simulink library "FirGeneric"  (R2022b)
settings: Solver=VariableStepAuto  StartTime=0.0  StopTime=10.0  RelTol=1e-3
undefined symbols (not defined in the file or in its folder): Row
libraries: HandyTextFile x9, TuneVar x9, FeaturePath x3, $bdroot x2, TOP x2, RTC x1
settings Model: Creator=fz1054048  LastModifiedBy=jk1043656

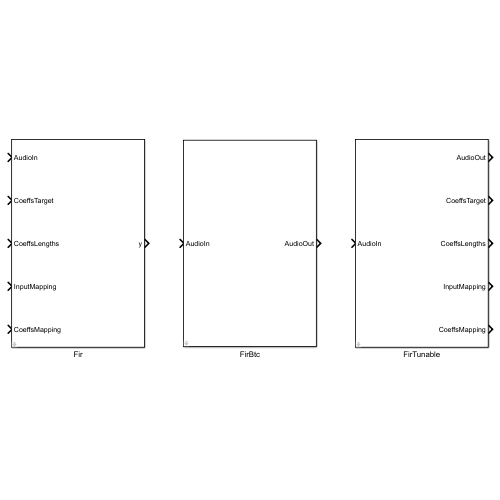
[thumbnail: Simulink's stored preview of the top-level diagram]
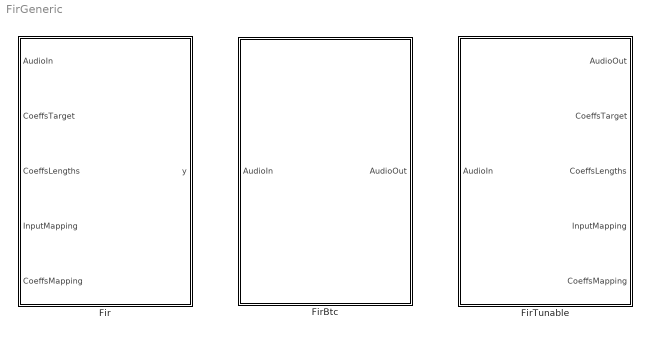
== system FirGeneric ==
  Fir : Subsystem  mask(Blocklib Fir){Config=[], FeatureName=Fir}
      mask prompts: Config "FirConfig"; FeatureName "Feature path name:"
      mask help:
      | For more information, see 'Help'. or run
      | >> help FirConfig
      mask init:
      | blkh=gcbh;
      | Config=BTConfig.Assert(blkh,Config);
      | 
      | Config.Validate();
      | Config.DoMaskInit(blkh);
      mask Help: eval("help FirConfig")
      mask TypeOptions FeatureName: FeaturePath/FeatureName
  FirBtc : Subsystem  mask(Blocklib FirBtc){Config=[], FeatureName=FirBtc}
      mask prompts: Config "FirBtcConfig"; FeatureName "Feature path name:"
      mask help:
      | For more information, see "Help" or run
      | >> help FirBtcConfig
      mask init:
      | blkh=gcbh;
      | Config=BTConfig.Assert(blkh,Config);
      | 
      | Config.Validate();
      | Config.DoMaskInit(blkh);
      mask Help: eval("help FirBtcConfig")
      mask TypeOptions FeatureName: FeaturePath/FeatureName
  FirTunable : Subsystem  mask(Blocklib FirTunable){Config=[], FeatureName=FirTunable}
      mask prompts: Config "FirTunableConfig"; FeatureName "Feature path name:"
      mask help:
      | For more information, see "Help" or run
      | >> help FirConfig
      mask init:
      | blkh=gcbh;
      | Config=BTConfig.Assert(blkh,Config);
      | 
      | Config.Validate();
      | Config.DoMaskInit(blkh);
      mask Help: eval("help FirConfig")
      mask TypeOptions FeatureName: FeaturePath/FeatureName

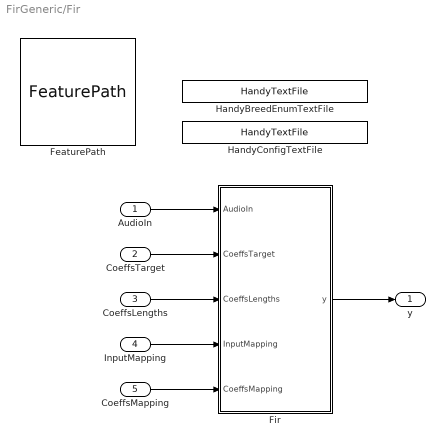
== system FirGeneric/Fir ==
  AudioIn : Inport
  CoeffsTarget : Inport  Port=2
  CoeffsLengths : Inport  Port=3
  InputMapping : Inport  Port=4
  CoeffsMapping : Inport  Port=5
  FeaturePath : FeaturePath/FeaturePath  FeatureName=Fir  IsGroup=off  GroupNumber=-1  IsModule=off  TriggerInit=[-5 -21 110 86]
      settings: SourceProductName=Bose Talaria
  Fir : Subsystem  Variant=on
  HandyBreedEnumTextFile : HandyTextFile/HandyTextFile  TemplateSource=<dialog fields>  FileSuffix=BreedEnum  OpenDialogOnLoad=off  UseThisBlockName=off  AddGrandParentNamePrefix=off  TheDefaultText=% $(FILENAME) $(PREFIX) $(SUFFIX)  ShowInLibBrowser=on
      settings: SourceProductName=Bose Talaria
  HandyConfigTextFile : HandyTextFile/HandyTextFile  TemplateSource=Config  FileSuffix=File  OpenDialogOnLoad=off  UseThisBlockName=off  AddGrandParentNamePrefix=off  TheDefaultText=% $(FILENAME) $(PREFIX) $(SUFFIX)  ShowInLibBrowser=on
      settings: SourceProductName=Bose Talaria
  y : Outport
  wires:
  AudioIn/1 -> Fir/1(AudioIn)
  CoeffsLengths/1 -> Fir/3(CoeffsLengths)
  InputMapping/1 -> Fir/4(InputMapping)
  CoeffsMapping/1 -> Fir/5(CoeffsMapping)
  Fir/1(y) -> y/1
  CoeffsTarget/1 -> Fir/2(CoeffsTarget)

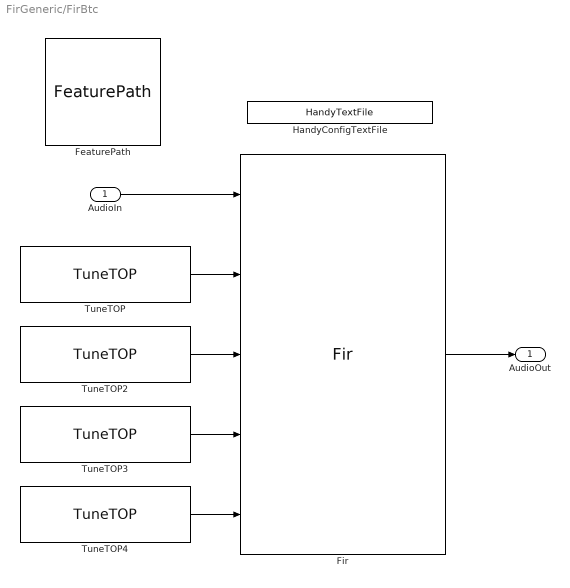
== system FirGeneric/FirBtc ==
  AudioIn : Inport
  FeaturePath : FeaturePath/FeaturePath  FeatureName=FirBtc  IsGroup=off  GroupNumber=-1  IsModule=off  TriggerInit=[-35 -26 80 81]
      settings: SourceProductName=Bose Talaria
  Fir : $bdroot/Fir  Config=Config  FeatureName=Fir
  HandyConfigTextFile : HandyTextFile/HandyTextFile  TemplateSource=Config  FileSuffix=File  OpenDialogOnLoad=off  UseThisBlockName=off  AddGrandParentNamePrefix=off  TheDefaultText=% $(FILENAME) $(PREFIX) $(SUFFIX)  ShowInLibBrowser=on
      settings: SourceProductName=Bose Talaria
  TuneTOP : TuneVar/TuneTOP  TriggerInit=[-60 182 110 238]  TopName=CoeffsTarget  TuneName=CoeffsTarget  DataTypeOut=single  TunabilityNumber=1  MinValue=[]  MaxValue=[]  BankNumber=Config.BankNumber  PreOverlay=false  PostOverlay=Config.PostOverlayRequired  UseSameName=on  MaskValue=Config.TuneVarCoeffsTarget
      settings: SourceProductName=Bose Talaria
  TuneTOP2 : TuneVar/TuneTOP  TriggerInit=[-60 262 110 318]  TopName=CoeffsLengths  TuneName=CoeffsLengths  DataTypeOut=uint32  TunabilityNumber=1  MinValue=[]  MaxValue=[]  BankNumber=0  PreOverlay=false  PostOverlay=Config.PostOverlayRequired  UseSameName=on  MaskValue=Config.TuneVarCoeffsLengths
      settings: SourceProductName=Bose Talaria
  TuneTOP3 : TuneVar/TuneTOP  TriggerInit=[-60 342 110 398]  TopName=InputMapping  TuneName=InputMapping  DataTypeOut=uint32  TunabilityNumber=1  MinValue=[]  MaxValue=[]  BankNumber=0  PreOverlay=false  PostOverlay=Config.PostOverlayRequired  UseSameName=on  MaskValue=Config.TuneVarInputMapping
      settings: SourceProductName=Bose Talaria
  TuneTOP4 : TuneVar/TuneTOP  TriggerInit=[-60 422 110 478]  TopName=CoeffsMapping  TuneName=CoeffsMapping  DataTypeOut=uint32  TunabilityNumber=1  MinValue=[]  MaxValue=[]  BankNumber=0  PreOverlay=false  PostOverlay=Config.PostOverlayRequired  UseSameName=on  MaskValue=Config.TuneVarCoeffsMapping
      settings: SourceProductName=Bose Talaria
  AudioOut : Outport
  wires:
  Fir/1 -> AudioOut/1
  TuneTOP4/1 -> Fir/5
  AudioIn/1 -> Fir/1
  TuneTOP/1 -> Fir/2
  TuneTOP2/1 -> Fir/3
  TuneTOP3/1 -> Fir/4

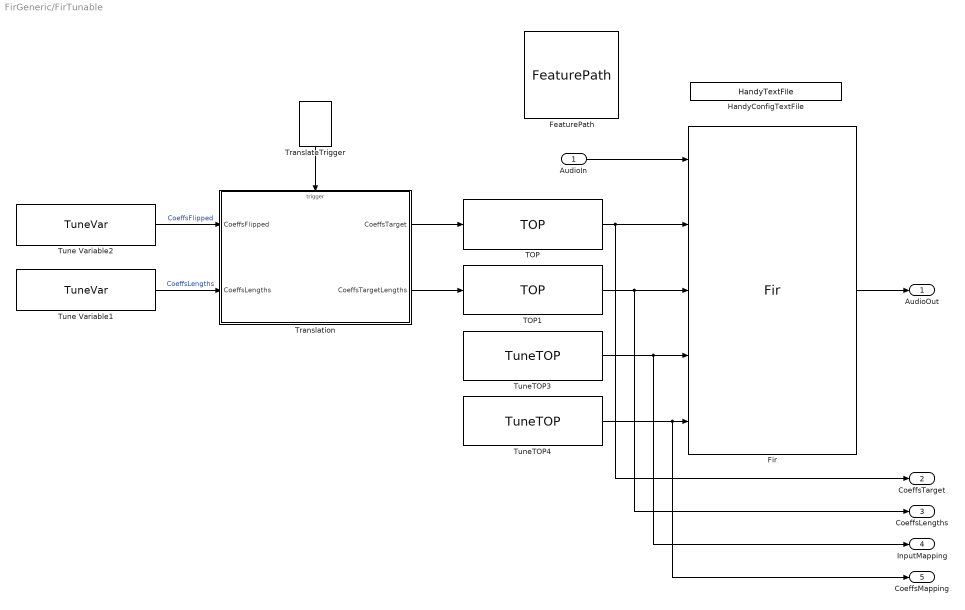
== system FirGeneric/FirTunable ==
  AudioIn : Inport
  FeaturePath : FeaturePath/FeaturePath  FeatureName=FirTunable  IsGroup=off  GroupNumber=-1  IsModule=off  TriggerInit=[-35 -26 80 81]
      settings: SourceProductName=Bose Talaria
  Fir : $bdroot/Fir  Config=Config  FeatureName=Fir
  HandyConfigTextFile : HandyTextFile/HandyTextFile  TemplateSource=Config  FileSuffix=File  OpenDialogOnLoad=off  UseThisBlockName=off  AddGrandParentNamePrefix=off  TheDefaultText=% $(FILENAME) $(PREFIX) $(SUFFIX)  ShowInLibBrowser=on
      settings: SourceProductName=Bose Talaria
  TOP : TOP/TOP  TriggerInit=[-110 180 60 240]  TopName=CoeffsTarget  DataTypeOut=single  BankNumber=Config.BankNumber  PreOverlay=false  PostOverlay=Config.PostOverlayRequired  CompatibilityString=Config.Breed  Role=Automatic
      settings: SourceProductName=Bose Talaria
  TOP1 : TOP/TOP  TriggerInit=[-110 260 60 320]  TopName=CoeffsLengths  DataTypeOut=uint32  BankNumber=0  PreOverlay=false  PostOverlay=Config.PostOverlayRequired  CompatibilityString=Config.Breed  Role=Automatic
      settings: SourceProductName=Bose Talaria
  TranslateTrigger : TuneVar/TranslateTrigger  TriggerInit=[-309 60 -271 115]
      settings: SourceProductName=Bose Talaria
  Translation : MATLAB Function  TreatAsAtomicUnit=on  mask{Breed=Config.Breed, FrameSize=Config.FrameSize, MaxAvgCoeffLength=Config.MaxAvgCoeffLength, NumFilters=Config.NumFilters}
  Tune Variable1 : TuneVar/TuneVar  TuneName=CoeffsLengths  SpecifyMaxSize=off  VariableDim=1 (Row)  MaxSize=[1 1]  TunabilityNumber=1  MinValue=[]  MaxValue=[]  TriggerInit=[-655 265 -485 315]  MaskValue=Config.TuneVarCoeffsLengths
      settings: SourceProductName=Bose Talaria
  Tune Variable2 : TuneVar/TuneVar  TuneName=CoeffsFlipped  SpecifyMaxSize=on  VariableDim=1 (Row)  MaxSize=[Config.MaxAvgCoeffLength*Config.NumFilters,1]  TunabilityNumber=1  MinValue=[]  MaxValue=[]  TriggerInit=[-655 185 -485 235]  MaskValue=Config.TuneVarCoeffsFlipped
      settings: SourceProductName=Bose Talaria
  TuneTOP3 : TuneVar/TuneTOP  TriggerInit=[-110 340 60 400]  TopName=InputMapping  TuneName=InputMapping  DataTypeOut=uint32  TunabilityNumber=1  MinValue=[]  MaxValue=[]  BankNumber=0  PreOverlay=false  PostOverlay=Config.PostOverlayRequired  UseSameName=on  MaskValue=Config.TuneVarInputMapping
      settings: SourceProductName=Bose Talaria
  TuneTOP4 : TuneVar/TuneTOP  TriggerInit=[-110 420 60 480]  TopName=CoeffsMapping  TuneName=CoeffsMapping  DataTypeOut=uint32  TunabilityNumber=1  MinValue=[]  MaxValue=[]  BankNumber=0  PreOverlay=false  PostOverlay=Config.PostOverlayRequired  UseSameName=on  MaskValue=Config.TuneVarCoeffsMapping
      settings: SourceProductName=Bose Talaria
  AudioOut : Outport
  CoeffsTarget : Outport  Port=2
  CoeffsLengths : Outport  Port=3
  InputMapping : Outport  Port=4
  CoeffsMapping : Outport  Port=5
  wires:
  TuneTOP3/1 -> Fir/4, InputMapping/1
  AudioIn/1 -> Fir/1
  TuneTOP4/1 -> Fir/5, CoeffsMapping/1
  Fir/1 -> AudioOut/1
  Translation/2(CoeffsTargetLengths) -> TOP1/1
  TranslateTrigger/1 -> Translation/Trigger
  Tune Variable1/1 -> Translation/2(CoeffsLengths)  "CoeffsLengths"
  Translation/1(CoeffsTarget) -> TOP/1
  Tune Variable2/1 -> Translation/1(CoeffsFlipped)  "CoeffsFlipped"
  TOP1/1 -> Fir/3, CoeffsLengths/1
  TOP/1 -> Fir/2, CoeffsTarget/1

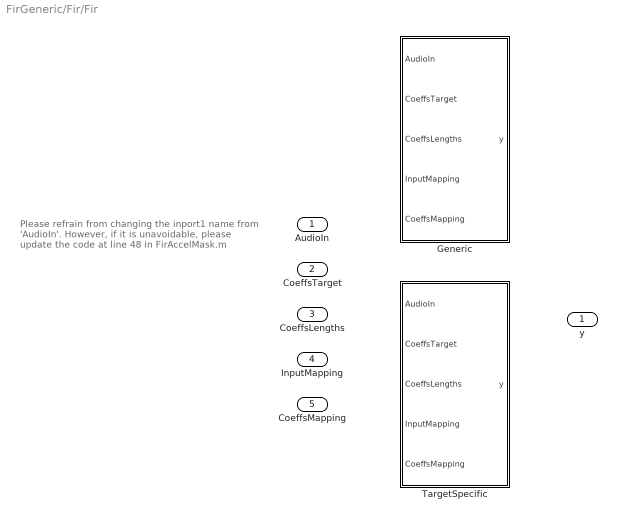
== system FirGeneric/Fir/Fir ==
  note: Please refrain from changing the inport1
      | name from 'AudioIn'. However, if it is
      | unavoidable, please update the code at
      | line 48 in FirAccelMask.m
  AudioIn : Inport
  CoeffsTarget : Inport  Port=2
  CoeffsLengths : Inport  Port=3
  InputMapping : Inport  Port=4
  CoeffsMapping : Inport  Port=5
  Generic : Subsystem  VariantControl=(Config.Breed == AsdHwEnum.Generic)
  TargetSpecific : Subsystem  VariantControl=(default)
  y : Outport

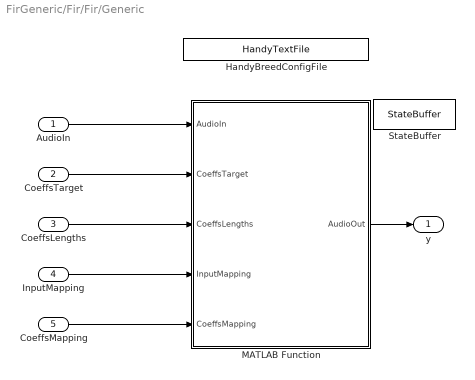
== system FirGeneric/Fir/Fir/Generic ==
  AudioIn : Inport
  CoeffsTarget : Inport  Port=2
  CoeffsLengths : Inport  Port=3
  InputMapping : Inport  Port=4
  CoeffsMapping : Inport  Port=5
  HandyBreedConfigFile : HandyTextFile/HandyTextFile  TemplateSource=<dialog fields>  FileSuffix=BreedConfig  OpenDialogOnLoad=off  UseThisBlockName=off  AddGrandParentNamePrefix=on  TheDefaultText=|  ShowInLibBrowser=on
      | % $(FILENAME) Setup model parameters for each "Init" callback (e.g. update diagram)
      | sample_rate_in_hertz = 44100;
      | frame_size = 32;
      | sysin_channel_count = 2;
      settings: SourceProductName=Bose Talaria
  MATLAB Function : MATLAB Function  TreatAsAtomicUnit=on  mask{FrameSize=Config.FrameSize, NumOutputs=Config.NumOutputs}
  StateBuffer : DataStoreMemory  DataStoreName=StateBuffer  WriteAfterWriteMsg=warning  InitialValue=single(zeros(Config.BreedObj.StateBufferSize,1))  ShowAdditionalParam=off  OutDataTypeStr=single
  y : Outport
  wires:
  AudioIn/1 -> MATLAB Function/1(AudioIn)
  CoeffsTarget/1 -> MATLAB Function/2(CoeffsTarget)
  CoeffsLengths/1 -> MATLAB Function/3(CoeffsLengths)
  InputMapping/1 -> MATLAB Function/4(InputMapping)
  CoeffsMapping/1 -> MATLAB Function/5(CoeffsMapping)
  MATLAB Function/1(AudioOut) -> y/1

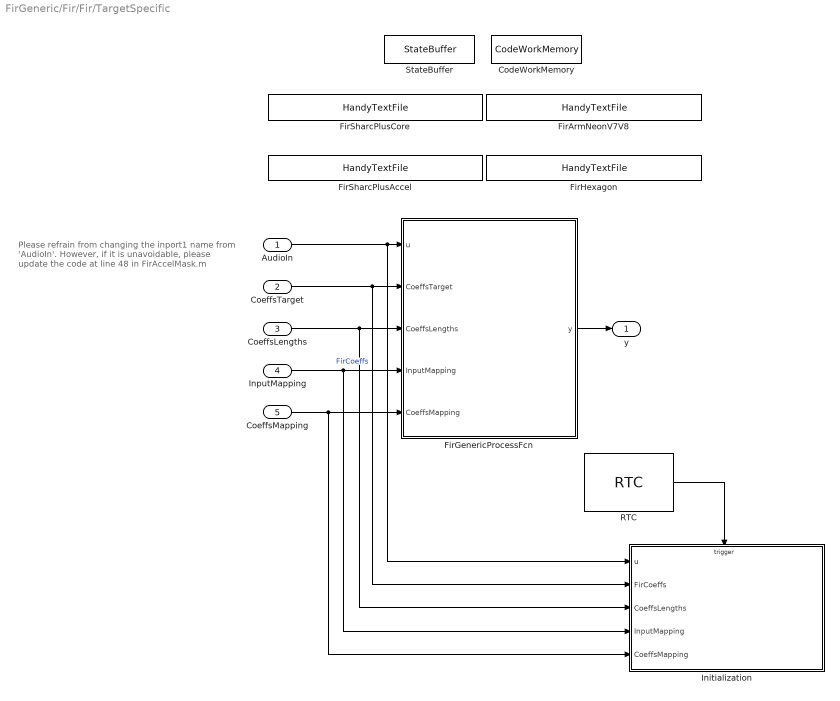
== system FirGeneric/Fir/Fir/TargetSpecific ==
  note: Please refrain from changing the inport1
      | name from 'AudioIn'. However, if it is
      | unavoidable, please update the code at
      | line 48 in FirAccelMask.m
  AudioIn : Inport
  CoeffsTarget : Inport  Port=2
  CoeffsLengths : Inport  Port=3
  InputMapping : Inport  Port=4
  CoeffsMapping : Inport  Port=5
  CodeWorkMemory : DataStoreMemory  DataStoreName=CodeWorkMemory  WriteAfterWriteMsg=warning  InitialValue=uint32(zeros(1,Config.BreedObj.CodeWorkMemorySize))  ShowAdditionalParam=off  OutDataTypeStr=uint32
  FirArmNeonV7V8 : HandyTextFile/HandyTextFile  TemplateSource=<dialog fields>  FileSuffix=BreedConfig  OpenDialogOnLoad=off  UseThisBlockName=on  AddGrandParentNamePrefix=off  TheDefaultText=|  ShowInLibBrowser=on
      | % $(FILENAME) Setup model parameters for each "Init" callback (e.g. update diagram)
      | sample_rate_in_hertz = 44100;
      | frame_size = 32;
      | sysin_channel_count = 2;
      settings: SourceProductName=Bose Talaria
  FirGenericProcessFcn : MATLAB Function  TreatAsAtomicUnit=on  mask{StateBufferSizeSimulation=Config.StateBufferSizeSimulation, Breed=Config.Breed}
  FirHexagon : HandyTextFile/HandyTextFile  TemplateSource=<dialog fields>  FileSuffix=BreedConfig  OpenDialogOnLoad=off  UseThisBlockName=on  AddGrandParentNamePrefix=off  TheDefaultText=|  ShowInLibBrowser=on
      | % $(FILENAME) Setup model parameters for each "Init" callback (e.g. update diagram)
      | sample_rate_in_hertz = 44100;
      | frame_size = 32;
      | sysin_channel_count = 2;
      settings: SourceProductName=Bose Talaria
  FirSharcPlusAccel : HandyTextFile/HandyTextFile  TemplateSource=<dialog fields>  FileSuffix=BreedConfig  OpenDialogOnLoad=off  UseThisBlockName=on  AddGrandParentNamePrefix=off  TheDefaultText=|  ShowInLibBrowser=on
      | % $(FILENAME) Setup model parameters for each "Init" callback (e.g. update diagram)
      | sample_rate_in_hertz = 44100;
      | frame_size = 32;
      | sysin_channel_count = 2;
      settings: SourceProductName=Bose Talaria
  FirSharcPlusCore : HandyTextFile/HandyTextFile  TemplateSource=<dialog fields>  FileSuffix=BreedConfig  OpenDialogOnLoad=off  UseThisBlockName=on  AddGrandParentNamePrefix=off  TheDefaultText=|  ShowInLibBrowser=on
      | % $(FILENAME) Setup model parameters for each "Init" callback (e.g. update diagram)
      | sample_rate_in_hertz = 44100;
      | frame_size = 32;
      | sysin_channel_count = 2;
      settings: SourceProductName=Bose Talaria
  Initialization : Subsystem
  RTC : RTC/RTC  REQ_Priority=RTC_Mask.NormalPriority  RequestAtInit=on  EnableRequest=on  REQElemType1=boolean  REQElemWidth1=1  REQElemInitial1=[]  REQElemType2=uint32  REQElemWidth2=1  REQElemInitial2=[]  REQElemType3=uint32  REQElemWidth3=1  REQElemInitial3=[]  REQElemType4=uint32  REQElemWidth4=1  REQElemInitial4=[]  REQElemType5=uint32  REQElemWidth5=1  REQElemInitial5=[]  REQElemType6=uint32  REQElemWidth6=1  REQElemInitial6=[]  REQElemType7=uint32  REQElemWidth7=1  REQElemInitial7=[]  REQElemType8=uint32  REQElemWidth8=1  REQElemInitial8=[]  REQElemType9=uint32  REQElemWidth9=1  REQElemInitial9=[]  REQElemType10=uint32  REQElemWidth10=1  REQElemInitial10=[]  EnableResponse=off  EnableRSP_StatusIn=off  RSPElemType1=uint32  RSPElemWidth1=1  RSPElemType2=uint32  RSPElemWidth2=1  RSPElemType3=uint32  RSPElemWidth3=1  RSPElemType4=uint32  RSPElemWidth4=1  RSPElemType5=uint32  RSPElemWidth5=1  RSPElemType6=uint32  RSPElemWidth6=1  RSPElemType7=uint32  RSPElemWidth7=1  RSPElemType8=uint32  RSPElemWidth8=1  RSPElemType9=uint32  RSPElemWidth9=1  RSPElemType10=uint32  RSPElemWidth10=1  EnableNotification=off  EnableNTF_PrepTrig=off  NTFElemType1=uint32  NTFElemWidth1=1  NTFElemType2=uint32  NTFElemWidth2=1  NTFElemType3=uint32  NTFElemWidth3=1  NTFElemType4=uint32  NTFElemWidth4=1  NTFElemType5=uint32  NTFElemWidth5=1  NTFElemType6=uint32  NTFElemWidth6=1  NTFElemType7=uint32  NTFElemWidth7=1  NTFElemType8=uint32  NTFElemWidth8=1  NTFElemType9=uint32  NTFElemWidth9=1  NTFElemType10=uint32  NTFElemWidth10=1  MaskMessageName=InitReset
      settings: SourceProductName=Bose Talaria
  StateBuffer : DataStoreMemory  DataStoreName=StateBuffer  WriteAfterWriteMsg=warning  InitialValue=single(zeros(Config.BreedObj.StateBufferSize,1))  ShowAdditionalParam=off  OutDataTypeStr=single
  y : Outport
  wires:
  FirGenericProcessFcn/1(y) -> y/1
  CoeffsTarget/1 -> Initialization/2(FirCoeffs), FirGenericProcessFcn/2(CoeffsTarget)  "FirCoeffs"
  RTC/1 -> Initialization/Trigger
  CoeffsMapping/1 -> Initialization/5(CoeffsMapping), FirGenericProcessFcn/5(CoeffsMapping)
  AudioIn/1 -> Initialization/1(u), FirGenericProcessFcn/1(u)
  InputMapping/1 -> Initialization/4(InputMapping), FirGenericProcessFcn/4(InputMapping)
  CoeffsLengths/1 -> Initialization/3(CoeffsLengths), FirGenericProcessFcn/3(CoeffsLengths)

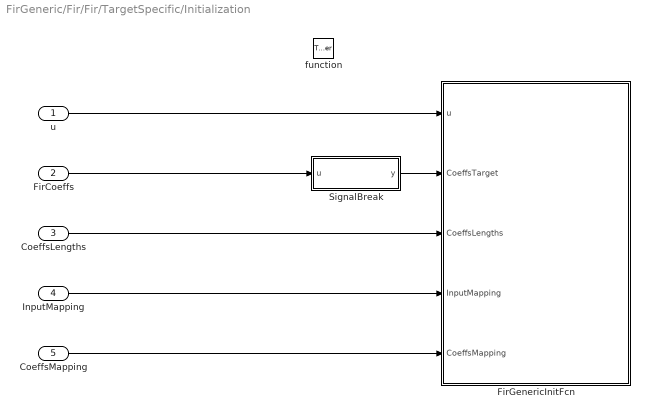
== system FirGeneric/Fir/Fir/TargetSpecific/Initialization ==
  u : Inport
  FirCoeffs : Inport  Port=2
  CoeffsLengths : Inport  Port=3
  InputMapping : Inport  Port=4
  CoeffsMapping : Inport  Port=5
  function : TriggerPort  TriggerType=function-call  VariantControl=(inherit)
  FirGenericInitFcn : MATLAB Function  TreatAsAtomicUnit=on  mask{Breed=Config.Breed}
  SignalBreak : Subsystem  Variant=on  VariantControl=Choice
  wires:
  InputMapping/1 -> FirGenericInitFcn/4(InputMapping)
  SignalBreak/1(y) -> FirGenericInitFcn/2(CoeffsTarget)
  CoeffsMapping/1 -> FirGenericInitFcn/5(CoeffsMapping)
  FirCoeffs/1 -> SignalBreak/1(u)
  CoeffsLengths/1 -> FirGenericInitFcn/3(CoeffsLengths)
  u/1 -> FirGenericInitFcn/1(u)

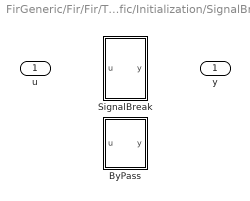
== system FirGeneric/Fir/Fir/TargetSpecific/Initialization/SignalBreak ==
  u : Inport
  ByPass : Subsystem  VariantControl=(default)
  SignalBreak : Subsystem  VariantControl=Config.Breed == AsdHwEnum.Hexagon
  y : Outport

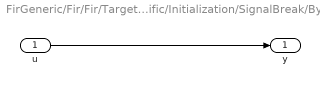
== system FirGeneric/Fir/Fir/TargetSpecific/Initialization/SignalBreak/ByPass ==
  u : Inport
  y : Outport
  wires:
  u/1 -> y/1

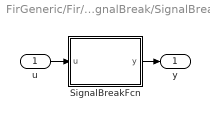
== system FirGeneric/Fir/Fir/TargetSpecific/Initialization/SignalBreak/SignalBreak ==
  u : Inport
  SignalBreakFcn : MATLAB Function  TreatAsAtomicUnit=on
  y : Outport
  wires:
  u/1 -> SignalBreakFcn/1(u)
  SignalBreakFcn/1(y) -> y/1

== matlab function FirGeneric/FirTunable/Translation ==
  data: CoeffsFlipped input; CoeffsLengths input; CoeffsTarget output; CoeffsTargetLengths output; Breed parameter; FrameSize parameter; MaxAvgCoeffLength parameter; NumFilters parameter
  events: trigger input FUNCTION_CALL_EVENT
function [CoeffsTarget, CoeffsTargetLengths] = FirTranslationMfb(CoeffsFlipped, CoeffsLengths, Breed, FrameSize, MaxAvgCoeffLength, NumFilters)
IsCoeffsRawFlipped = true;                          % Assume Coefficients are already flipped

% Check that CoeffsLengths don't exceed Maximum specified
if sum(CoeffsLengths.Value) > NumFilters*MaxAvgCoeffLength
    TranslateError('Length of Coefficients of specified by CoeffsLengths should not be greater than NumFilters*MaxAvgCoeffLength');
end

% Check that CoeffsLengths and CoeffsRaw are appropriately sized.
if numel(CoeffsFlipped.Value) < sum(CoeffsLengths.Value)
    TranslateError('Number of all coefficients in CoeffsFlipped should be greater than or equal to the sum of CoeffsLengths.');
end

[CoeffsTarget, CoeffsTargetLengths] = FirTranslation( ...
    single(CoeffsFlipped.Value), ...
    uint32(CoeffsLengths.Value),...
    Breed,...
    NumFilters,...
    MaxAvgCoeffLength,...
    FrameSize,...
    IsCoeffsRawFlipped);
end

== matlab function FirGeneric/Fir/Fir/Generic/MATLAB Function ==
  data: AudioIn input; AudioOut output; CoeffsTarget input; CoeffsLengths input; InputMapping input; CoeffsMapping input; FrameSize parameter; NumOutputs parameter; StateBuffer data_store_memory
function AudioOut = FirGenericProcess(AudioIn, CoeffsTarget, CoeffsLengths, InputMapping, CoeffsMapping, FrameSize, NumOutputs)
global StateBuffer;

NumOutputs = numel(CoeffsMapping);
AudioOut = FirGenericProcessSim(AudioIn, CoeffsTarget, numel(StateBuffer), CoeffsLengths, ...
                InputMapping, CoeffsMapping, FrameSize, NumOutputs);
end

== matlab function FirGeneric/Fir/Fir/TargetSpecific/Initialization/FirGenericInitFcn ==
  data: u input; CoeffsTarget input; CoeffsLengths input; InputMapping input; CoeffsMapping input; Breed parameter; CodeWorkMemory data_store_memory; StateBuffer data_store_memory
  function FirGenericInit(u, CoeffsTarget, CoeffsLengths, InputMapping, CoeffsMapping, Breed)
% Generic FIR function to work with M inputs, N outputs and K filters
%
% Parameters:
%   u:              input channels [frame size x number of inputs]
%   CoeffsTarget:    coefficient sets [total filter lengths x 1]
%   CoeffsLengths:  array of filter lengths [number of filters x 1]
%   InputMapping:   zero-based input mapping for each filter  [number of outputs x 1]
%   CoeffsMapping:  zero-based filter mapping for each filter [number of outputs x 1]
%
% Global parameters:
%   States:         array of states [totalBufferSize x 1]
%   CodeWorkMemory: working memory set up during roommode reset/init CRL
%                   function call [codeWorkMemorySize x 1]
%--------------------------------------------------------------------------

% Extract configuration information from inputs
[FrameSize, NumInputs]  = size(u);
NumOutputs = numel(InputMapping);

global StateBuffer;
global CodeWorkMemory;

% Get the work memory and states size
WorkMemorySize = numel(CodeWorkMemory);
StateBufferSize = numel(StateBuffer);

% Set correct data types
CoeffsLengths = uint32(CoeffsLengths);
NumCoeffSets = uint32(numel(CoeffsLengths));
FrameSize = uint32(FrameSize);
NumOutputs = uint32(NumOutputs);
NumInputs = uint32(NumInputs);
WorkMemorySize = uint32(WorkMemorySize);
StateBufferSize = uint32(StateBufferSize);

switch(Breed)
    case {AsdHwEnum.SharcPlusCore}
        y = fir_core_init(u, CoeffsTarget, StateBuffer, CoeffsLengths, InputMapping, CoeffsMapping, ...
            FrameSize, NumCoeffSets, NumInputs, NumOutputs, CodeWorkMemory);
        CodeWorkMemory(1) = y;
        
    case {AsdHwEnum.SharcPlusAccel}
        y = fir_accelerator_init(u, CoeffsTarget, StateBuffer, StateBufferSize, CoeffsLengths, InputMapping, ...
            CoeffsMapping, FrameSize, NumCoeffSets, NumInputs, NumOutputs, ...
            CodeWorkMemory, WorkMemorySize);
        CodeWorkMemory(1) = y;

    case {AsdHwEnum.Hexagon}
        y = fir_hexagon_init(u, CoeffsTarget, StateBuffer, CoeffsLengths, InputMapping, CoeffsMapping, ...
            FrameSize, NumCoeffSets, NumInputs, NumOutputs, CodeWorkMemory);
        CodeWorkMemory(1) = y;
            
    case {AsdHwEnum.ArmNeonV7V8}
        y = fir_armv7v8_init(u, CoeffsTarget, StateBuffer, CoeffsLengths, InputMapping, CoeffsMapping, ...
            FrameSize, NumCoeffSets, NumInputs, NumOutputs, CodeWorkMemory);
        CodeWorkMemory(1) = y;

end

end


function y = fir_accelerator_init(u, coeffs, states, statesSize, CoeffsLengths, inputMapping, CoeffsMapping,...
                                  frameSize, numCoeffSets, numInputs, numOutputs, workMemory,...
                                  workMemorySize)                         
% If target == codegen, error out if no CRL found
coder.replace('-errorifnoreplacement');

% No init simulation code, but need to do something to ensure CRL does not
% get optimized out
y = workMemory(1) + 1;

end

function y = fir_core_init(u, coeffs, states, CoeffsLengths, inputMapping, CoeffsMapping,...
                             frameSize, numCoeffSets, numInputs, numOutputs, workMemory)
% If target == codegen, error out if no CRL found
coder.replace('-errorifnoreplacement');

% No init simulation code, but need to do something to ensure CRL does not
% get optimized out
y = workMemory(1) + 1;

end


function y = fir_hexagon_init(u, coeffs, states, CoeffsLengths, inputMapping, CoeffsMapping,...
                             frameSize, numCoeffSets, numInputs, numOutputs, workMemory)
% If target == codegen, error out if no CRL found
coder.replace('-errorifnoreplacement');

% No init simulation code, but need to do something to ensure CRL does not
% get optimized out
y = workMemory(1) + 1;

end

function y = fir_armv7v8_init(u, coeffs, states, CoeffsLengths, inputMapping, CoeffsMapping,...
                             frameSize, numCoeffSets, numInputs, numOutputs, workMemory)
% If target == codegen, error out if no CRL found
coder.replace('-errorifnoreplacement');

% No init simulation code, but need to do something to ensure CRL does not
% get optimized out
y = workMemory(1) + 1;

end

== matlab function FirGeneric/Fir/Fir/TargetSpecific/FirGenericProcessFcn ==
  data: u input; CoeffsTarget input; y output; CoeffsLengths input; InputMapping input; CoeffsMapping input; Breed parameter; CodeWorkMemory data_store_memory; StateBufferSizeSimulation parameter
function y = FirGenericProcess(u, CoeffsTarget, CoeffsLengths, InputMapping, CoeffsMapping, Breed, StateBufferSizeSimulation)
% Generic FIR function to work with M inputs, N outputs and K filters
%
% Parameters:
%   u:              input channels [frame size x number of inputs]
%   CoeffsTarget:   coefficient sets, translated to target specfic format [total filter lengths x 1]
%   CoeffsLengths:  array of filter lengths [number of filters x 1]
%   InputMapping:   zero-based input mapping for each filter  [number of outputs x 1]
%   CoeffsMapping:  zero-based filter mapping for each filter [number of outputs x 1]
%   Breed:          string corresponding to the breed type
%
% Global parameters:
%   States:         array of states [totalBufferSize x 1]
%   CodeWorkMemory: working memory set up during roommode reset/init CRL
%                   function call [codeWorkMemorySize x 1]
%--------------------------------------------------------------------------


% Extract configuration information from inputs
[FrameSize, ~]  = size(u);
NumOutputs = numel(InputMapping);

global CodeWorkMemory;

% Define persistent variables for SharcPlusAccel Breed
persistent DelayedOut;
    
% Set correct data types
CoeffsLengths = uint32(CoeffsLengths);
FrameSize = uint32(FrameSize);
NumOutputs = uint32(NumOutputs);
InputMapping = uint32(InputMapping);

% Simulation
if(coder.target('MATLAB') || coder.target('Sfun')) 
    switch(Breed)
        case {AsdHwEnum.SharcPlusAccel}
            % Define one-frame delay buffer only for Accelerator simulation 
            % Simulink will optimize this out for code generation
            if isempty(DelayedOut)
                DelayedOut = single(zeros(FrameSize, NumOutputs));
            end
            % Manually insert one-frame delay in simulation to mimic 
            % Accelerator behavior
            y = DelayedOut;
            DelayedOut = FirGenericProcessSim(u, CoeffsTarget, StateBufferSizeSimulation, CoeffsLengths, InputMapping, ...
                CoeffsMapping, FrameSize, NumOutputs, Breed);
        otherwise
            y = FirGenericProcessSim(u, CoeffsTarget, StateBufferSizeSimulation, CoeffsLengths, InputMapping, ...
                CoeffsMapping, FrameSize, NumOutputs, Breed);
    end
% Code Generation: same function prototype for core and accel
else
    switch(Breed)
        case {AsdHwEnum.SharcPlusCore}
            y = fir_core_process(u, CodeWorkMemory, NumOutputs);
        case {AsdHwEnum.SharcPlusAccel}
            y = fir_accelerator_process(u, CodeWorkMemory, NumOutputs);
        case {AsdHwEnum.Hexagon}
            y = fir_hexagon_process(u, CodeWorkMemory, NumOutputs);
        case {AsdHwEnum.ArmNeonV7V8}
            y = fir_armv7v8_process(single(u), uint32(CodeWorkMemory), uint32(NumOutputs));
    end
end
end

%% CRL functions for code generation
function y = fir_core_process(u, WorkMemory, NumOutputs)
% If target == codegen, error out if no CRL found
coder.replace('-errorifnoreplacement');
[FrameSize, ~]  = size(u);
y = single(zeros(FrameSize, NumOutputs));
end

function y = fir_accelerator_process(u, WorkMemory, NumOutputs)
% If target == codegen, error out if no CRL found
coder.replace('-errorifnoreplacement');
[FrameSize, ~]  = size(u);
y = single(zeros(FrameSize, NumOutputs));
end

function y = fir_hexagon_process(u, workMemory, numOutputs)
% If target == codegen, error out if no CRL found
coder.replace('-errorifnoreplacement');
[frameSize, ~]  = size(u);
y = single(zeros(frameSize, numOutputs));
end

function y = fir_armv7v8_process(u, workMemory, numOutputs)
% If target == codegen, error out if no CRL found
coder.replace('-errorifnoreplacement');
[frameSize, ~]  = size(u);
y = single(zeros(frameSize, numOutputs));
end

== matlab function FirGeneric/Fir/Fir/TargetSpecific/Initialization/SignalBreak/SignalBreak/SignalBreakFcn ==
  data: u input; y output
function y = fcn(u)

y = u;
